simulink model "newModel"  (R2015a)
settings: Solver=FixedStepDiscrete  StartTime=0.0  StopTime=1500  FixedStep=1  RelTol=1e-3
(part 2 of 2)

== stateflow chart newModel/receiver/detectMainFrame ==
  settings: executeAtInitialization=1  initializeOutput=1
  state detectMainFrame [parallel]
    settings: executionOrder=1
    state FIFO
      du:
      master = detectMainFrame(samples);
      FIFO -> FIFO : [clk==1]
          | {
          | samples  = BufferFIFO(samples, md);
          | }
  data: A function_input boolean size=144; c function_input boolean; r function_output boolean size=144; A function_input boolean size=144; r function_output boolean; samples local boolean size=144; m1front local boolean =0; m2front local boolean =0; m3front local boolean =0; m4front local boolean =0; m5front local boolean =0; m6front local boolean =0; m7front local boolean =0; m8front local boolean =0; m9front local boolean =0; m1back local boolean =0; m2back local boolean =0; m3back local boolean =0; m4back local boolean =0; m5back local boolean =0; m6back local boolean =0; m7back local boolean =0; m8back local boolean =0; m9back local boolean =0; md input boolean; master local boolean; clk input boolean
  data md settings: description=in
  data clk settings: description=in
  function r = BufferFIFO(A, c):
    | function r = BufferFIFO(A, c)
    | A(2:144) = A(1:143);
    | A(1) = c;
    | r = A;
  function r = detectMainFrame(A):
    | function r = detectMainFrame(A)
    | % start
    | % case samples(143 downto 136) is
    | %		       when"11111111"|"11111110"|"11111101"|"11111011"|"11110111"|"11101111"|"11011111"|"10111111"|"01111111"|"00111111"|"11111100"|"01111110"|"00111100"=>%
    | %			        m1front<='1';
    | %			    when others=>
    | %			        m1front<='0';
    | %		  end case;
    | %		  --检测帧起始符的后半部分
    | %		  case samples(135 downto 128)  is
    | %		       when "00000000"|"00000001"|"00000010"|"00000100"|"00001000"|"00010000"|"00100000"|"01000000"|"10000000"|"11000000"|"00000011"|"10000001"|"11000011"=>
    | %			        m1back<='1';
    | %			    when others=>
    | %			        m1back<='0';
    | %		  end case;
    | if (A(137)==1 && A(138)==1 && A(139)==1&& A(140)==1&& A(141)==1&& A(142)==1&& A(143)==1&& A(144)==1) || ...
    |     (A(137)==1 && A(138)==0 && A(139)==1&& A(140)==1&& A(141)==1&& A(142)==1&& A(143)==1&& A(144)==1) || ...
    |     (A(137)==1 && A(138)==1 && A(139)==0&& A(140)==1&& A(141)==1&& A(142)==1&& A(143)==1&& A(144)==1) || ...
    |     (A(137)==1 && A(138)==1 && A(139)==1&& A(140)==0&& A(141)==1&& A(142)==1&& A(143)==1&& A(144)==1) || ...
    |     (A(137)==1 && A(138)==1 && A(139)==1&& A(140)==1&& A(141)==0&& A(142)==1&& A(143)==1&& A(144)==1) || ...
    |     (A(137)==1 && A(138)==1 && A(139)==1&& A(140)==1&& A(141)==1&& A(142)==0&& A(143)==1&& A(144)==1) || ...
    |     (A(137)==1 && A(138)==1 && A(139)==1&& A(140)==1&& A(141)==1&& A(142)==1&& A(143)==0&& A(144)==1) || ...
    |     (A(137)==1 && A(138)==1 && A(139)==1&& A(140)==1&& A(141)==1&& A(142)==1&& A(143)==1&& A(144)==0) || ...
    |     (A(137)==1 && A(138)==1 && A(139)==1&& A(140)==1&& A(141)==1&& A(142)==1&& A(143)==0&& A(144)==0) || ...
    |     (A(137)==0 && A(138)==0 && A(139)==1&& A(140)==1&& A(141)==1&& A(142)==1&& A(143)==1&& A(144)==1) || ...
    |     (A(137)==0 && A(138)==1 && A(139)==1&& A(140)==1&& A(141)==1&& A(142)==1&& A(143)==1&& A(144)==0) || ...
    |     (A(137)==0 && A(138)==0 && A(139)==1&& A(140)==1&& A(141)==1&& A(142)==1&& A(143)==0&& A(144)==0)
    |     m1front = true;
    | else
    |     m1front = false;
    | end
    | if (A(129)==0 && A(130)==0 && A(131)==0 && A(132)==0 && A(133)==0 && A(134)==0&& A(135)==0&& A(136)==0) || ...
    |         (A(129)==0 && A(130)==0 && A(131)==0 && A(132)==0 && A(133)==0 && A(134)==0&& A(135)==0&& A(136)==1) || ...
    |         (A(129)==0 && A(130)==0 && A(131)==0 && A(132)==0 && A(133)==0 && A(134)==0&& A(135)==1&& A(136)==0) || ...
    |         (A(129)==0 && A(130)==0 && A(131)==0 && A(132)==0 && A(133)==0 && A(134)==1&& A(135)==0&& A(136)==0) || ...
    |         (A(129)==0 && A(130)==0 && A(131)==0 && A(132)==0 && A(133)==1 && A(134)==0&& A(135)==0&& A(136)==0) || ...
    |         (A(129)==0 && A(130)==0 && A(131)==0 && A(132)==1 && A(133)==0 && A(134)==0&& A(135)==0&& A(136)==0) || ...
    |         (A(129)==0 && A(130)==0 && A(131)==1 && A(132)==0 && A(133)==0 && A(134)==0&& A(135)==0&& A(136)==0) || ...
    |         (A(129)==0 && A(130)==1 && A(131)==0 && A(132)==0 && A(133)==0 && A(134)==0&& A(135)==0&& A(136)==0) || ...
    |         (A(129)==1 && A(130)==0 && A(131)==0 && A(132)==0 && A(133)==0 && A(134)==0&& A(135)==0&& A(136)==0) || ...
    |         (A(129)==1 && A(130)==1 && A(131)==0 && A(132)==0 && A(133)==0 && A(134)==0&& A(135)==0&& A(136)==0) || ...
    |         (A(129)==0 && A(130)==0 && A(131)==0 && A(132)==0 && A(133)==0 && A(134)==0&& A(135)==1&& A(136)==1) || ...
    |         (A(129)==1 && A(130)==0 && A(131)==0 && A(132)==0 && A(133)==0 && A(134)==0&& A(135)==0&& A(136)==1) || ...
    |         (A(129)==1 && A(130)==1 && A(131)==0 && A(132)==0 && A(133)==0 && A(134)==0&& A(135)==1&& A(136)==1)
    |     m1back = true;
    | else
    |     m1back = false;
    | end
    | %%%%%%%%%%%%%%%%%%%%%%%%%%%%%%%%%%%%%%%%%%%%%%%%%%%%%%%%%%%%%%%%%%%%%%%%%%%%%%%%%%%%%%%%%%%%%%%%%%%%%%%%%%%%%%%%%%%%%%%%%%%%%%%%%%%%%%%%%%%%%%%%%%%%%%
    | if A(124) == 1
    |     m2front = true;
    | else
    |     m2front = false;
    | end
    | if A(116) == 1
    |     m2back = true;
    | else
    |     m2back = false;
    | end
    | if A(108) == 0
    |     m3front = true;
    | else
    |     m3front = false;
    | end
    | if A(100) == 0
    |     m3back = true;
    | else
    |     m3back = false;
    | end
    | if A(92) == 0
    |     m4front = true;
    | else
    |     m4front = false;
    | end
    | if A(84) == 1
    |     m4back = true;
    | else
    |     m4back = false;
    | end
    | if A(76) == 1
    |     m5front = true ;
    | else
    |     m5front = false;
    | end
    | if A(68) == 1
    |     m5back = true;
    | else
    |     m5back = false;
    | end
    | if A(60) == 0
    |     m6front = true;
    | else
    |     m6front = false;
    | end
    | if A(52) == 0
    |     m6back = true;
    | else
    |     m6back = false;
    | end
    | if A(44) == 0
    |     m7front = true;
    | else
    |     m7front = false;
    | end
    | if A(36) == 1
    |     m7back = true;
    | else
    |     m7back = false;
    | end
    | if A(28) == 0
    |     m8front = true;
    | else
    |     m8front = false;
    | end
    | if A(20) == 1
    |     m8back = true;
    | else
    |     m8back = false;
    | end
    | if A(12) == 0
    |     m9front = true;
    | else
    |     m9front = false;
    | end
    | if A(4) == 1
    |     m9back = true;
    | else
    |     m9back = false;
    | end
    | r = m1front && m2front && m3front && m4front && m5front && m6front && m7front && m8front && m9front && m1back && m2back && m3back && m4back && m5back && m6back && m7back && m8back && m9back;

== stateflow chart newModel/receiver/detectSlaveFrame ==
  settings: executeAtInitialization=1  initializeOutput=1
  state detectSlaveFrame [parallel]
    settings: executionOrder=1
    state FIFO
      du:
      slave = detectSlaveFrame(samples);
      FIFO -> FIFO : [clk==1]
          | {
          | samples  = BufferFIFO(samples, md);
          | }
  data: A function_input boolean size=144; c function_input boolean; r function_output boolean size=144; A function_input boolean size=144; r function_output boolean; samples local boolean size=144; s1front local boolean =0; s2front local boolean =0; s3front local boolean =0; s4front local boolean =0; s5front local boolean =0; s6front local boolean =0; s7front local boolean =0; s8front local boolean =0; s9front local boolean =0; s1back local boolean =0; s2back local boolean =0; s3back local boolean =0; s4back local boolean =0; s5back local boolean =0; s6back local boolean =0; s7back local boolean =0; s8back local boolean =0; s9back local boolean =0; md input boolean; slave local boolean; clk input boolean
  data md settings: description=in
  data clk settings: description=in
  function r = BufferFIFO(A, c):
    | function r = BufferFIFO(A, c)
    | A(2:144) = A(1:143);
    | A(1) = c;
    | r = A;
  function r = detectSlaveFrame(A):
    | function r = detectSlaveFrame(A)
    | % start DetectSlave slave%%%%%%%%%%%%%%%%%%%%%%%%%%%%%%%%%%%%%%%%%%%%%%%%%%%%%%%%%%%%%%%%%%%%%%%%%%%%%%%%%%%%%%%%%%%%%%%%%%%%%%%%
    | if (A(137)==1 && A(138)==1 && A(139)==1&& A(140)==1&& A(141)==1&& A(142)==1&& A(143)==1&& A(144)==1) || ...
    |     (A(137)==1 && A(138)==0 && A(139)==1&& A(140)==1&& A(141)==1&& A(142)==1&& A(143)==1&& A(144)==1) || ...
    |     (A(137)==1 && A(138)==1 && A(139)==0&& A(140)==1&& A(141)==1&& A(142)==1&& A(143)==1&& A(144)==1) || ...
    |     (A(137)==1 && A(138)==1 && A(139)==1&& A(140)==0&& A(141)==1&& A(142)==1&& A(143)==1&& A(144)==1) || ...
    |     (A(137)==1 && A(138)==1 && A(139)==1&& A(140)==1&& A(141)==0&& A(142)==1&& A(143)==1&& A(144)==1) || ...
    |     (A(137)==1 && A(138)==1 && A(139)==1&& A(140)==1&& A(141)==1&& A(142)==0&& A(143)==1&& A(144)==1) || ...
    |     (A(137)==1 && A(138)==1 && A(139)==1&& A(140)==1&& A(141)==1&& A(142)==1&& A(143)==0&& A(144)==1) || ...
    |     (A(137)==1 && A(138)==1 && A(139)==1&& A(140)==1&& A(141)==1&& A(142)==1&& A(143)==1&& A(144)==0) || ...
    |     (A(137)==1 && A(138)==1 && A(139)==1&& A(140)==1&& A(141)==1&& A(142)==1&& A(143)==0&& A(144)==0) || ...
    |     (A(137)==0 && A(138)==0 && A(139)==1&& A(140)==1&& A(141)==1&& A(142)==1&& A(143)==1&& A(144)==1) || ...
    |     (A(137)==0 && A(138)==1 && A(139)==1&& A(140)==1&& A(141)==1&& A(142)==1&& A(143)==1&& A(144)==0) || ...
    |     (A(137)==0 && A(138)==0 && A(139)==1&& A(140)==1&& A(141)==1&& A(142)==1&& A(143)==0&& A(144)==0)
    |     s1front = true;
    | else
    |     s1front = false;
    | end
    | if (A(129)==0 && A(130)==0 && A(131)==0 && A(132)==0 && A(133)==0 && A(134)==0&& A(135)==0&& A(136)==0) || ...
    |         (A(129)==0 && A(130)==0 && A(131)==0 && A(132)==0 && A(133)==0 && A(134)==0&& A(135)==0&& A(136)==1) || ...
    |         (A(129)==0 && A(130)==0 && A(131)==0 && A(132)==0 && A(133)==0 && A(134)==0&& A(135)==1&& A(136)==0) || ...
    |         (A(129)==0 && A(130)==0 && A(131)==0 && A(132)==0 && A(133)==0 && A(134)==1&& A(135)==0&& A(136)==0) || ...
    |         (A(129)==0 && A(130)==0 && A(131)==0 && A(132)==0 && A(133)==1 && A(134)==0&& A(135)==0&& A(136)==0) || ...
    |         (A(129)==0 && A(130)==0 && A(131)==0 && A(132)==1 && A(133)==0 && A(134)==0&& A(135)==0&& A(136)==0) || ...
    |         (A(129)==0 && A(130)==0 && A(131)==1 && A(132)==0 && A(133)==0 && A(134)==0&& A(135)==0&& A(136)==0) || ...
    |         (A(129)==0 && A(130)==1 && A(131)==0 && A(132)==0 && A(133)==0 && A(134)==0&& A(135)==0&& A(136)==0) || ...
    |         (A(129)==1 && A(130)==0 && A(131)==0 && A(132)==0 && A(133)==0 && A(134)==0&& A(135)==0&& A(136)==0) || ...
    |         (A(129)==1 && A(130)==1 && A(131)==0 && A(132)==0 && A(133)==0 && A(134)==0&& A(135)==0&& A(136)==0) || ...
    |         (A(129)==0 && A(130)==0 && A(131)==0 && A(132)==0 && A(133)==0 && A(134)==0&& A(135)==1&& A(136)==1) || ...
    |         (A(129)==1 && A(130)==0 && A(131)==0 && A(132)==0 && A(133)==0 && A(134)==0&& A(135)==0&& A(136)==1) || ...
    |         (A(129)==1 && A(130)==1 && A(131)==0 && A(132)==0 && A(133)==0 && A(134)==0&& A(135)==1&& A(136)==1)
    |     s1back = true;
    | else
    |     s1back = false;
    | end
    | %%%%%%%%%%%%%%%%%%%%%%%%%%%%%%%%%%%%%%%%%%%%%%%%%%%%%%%%%%%%%%%%%%%%%%%%%%%%%%%%%%%%%%%%%%%%%%%%%%%%%%%%%%%%%%%%%%%%%%%%%%%%%%%%%%%%%%%%%%%%%
    | if A(124) == 1
    |     s2front = true;
    | else
    |     s2front = false;
    | end
    | if A(116) == 0
    |     s2back = true;
    | else
    |     s2back = false;
    | end
    | if A(108) == 1
    |     s3front = true;
    | else
    |     s3front = false;
    | end
    | if A(100) == 0
    |     s3back = true;
    | else
    |     s3back = false;
    | end
    | if A(92) == 1
    |     s4front = true;
    | else
    |     s4front = false;
    | end
    | if A(84) == 0
    |     s4back = true;
    | else
    |     s4back = false;
    | end
    | if A(76) == 0
    |     s5front = true ;
    | else
    |     s5front = false;
    | end
    | if A(68) == 0
    |     s5back = true;
    | else
    |     s5back = false;
    | end
    | if A(60) == 1
    |     s6front = true;
    | else
    |     s6front = false;
    | end
    | if A(52) == 1
    |     s6back = true;
    | else
    |     s6back = false;
    | end
    | if A(44) == 1
    |     s7front = true;
    | else
    |     s7front = false;
    | end
    | if A(36) == 0
    |     s7back = true;
    | else
    |     s7back = false;
    | end
    | if A(28) == 0
    |     s8front = true;
    | else
    |     s8front = false;
    | end
    | if A(20) == 0
    |     s8back = true;
    | else
    |     s8back = false;
    | end
    | if A(12) == 1
    |     s9front = true;
    | else
    |     s9front = false;
    | end
    | if A(4) == 1
    |     s9back = true;
    | else
    |     s9back = false;
    | end
    | r = s1front && s2front && s3front && s4front && s5front && s6front && s7front && s8front && s9front && s1back && s2back && s3back && s4back && s5back && s6back && s7back && s8back && s9back;

== stateflow chart newModel/receiver/or ==
  settings: executeAtInitialization=1  initializeOutput=1
  state or [parallel]
    settings: executionOrder=1
    state start
      du:
      start = master || slave;
    (default) -> start
  data: master input boolean; start local boolean; slave input boolean
